simulink model "DrivetrainEv_3motor"  (R2019b)
settings: configuration reference "Reference" (kept outside this file)
undefined symbols (not defined in the file): b, b_CG, br, g, k, Mass, Ndiff_rear, NF, NR, T
libraries: autolibshared x8, autolibsharedcoupling x5, autolibcoupling x2, autolibutils x2, autolibshareddiff x1
(part 1 of 4)
settings Model: DataDictionary=SystemDD.sldd  ModifiedByFormat=The MathWorks, Inc.  PauseTimes=10  Creator=The MathWorks, Inc.  LastModifiedBy=The MathWorks, Inc.
settings ConfigSetRef: SourceName=Reference

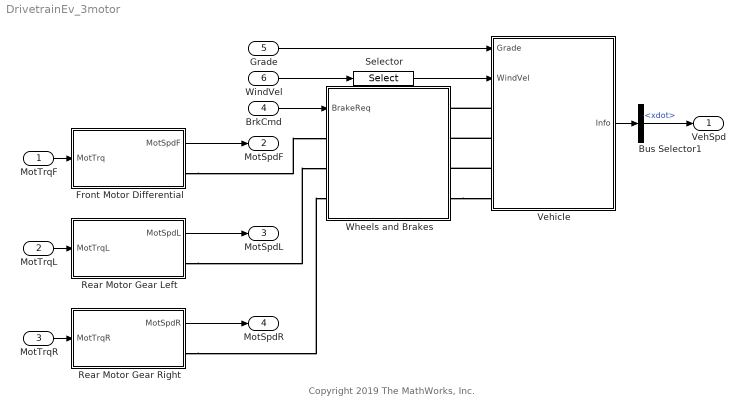
== system DrivetrainEv_3motor ==
  note: Copyright 2019 The MathWorks, Inc.
  MotTrqF : Inport
  MotTrqL : Inport  Port=2
  MotTrqR : Inport  Port=3
  BrkCmd : Inport  Port=4
  Grade : Inport  Port=5
  WindVel : Inport  Port=6
  Bus Selector1 : BusSelector  OutputSignals=BdyFrm.Cg.Vel.xdot
  Front Motor Differential : Subsystem  VariantControl=0
  Rear Motor Gear Left : Subsystem  VariantControl=0
  Rear Motor Gear Right : Subsystem  VariantControl=0
  Selector : Selector  InputPortWidth=3  IndexOptions=Index vector (dialog)  Indices=[1]  OutputSizes=1
  Vehicle : Subsystem
  Wheels and Brakes : Subsystem  VariantControlMode=Label  Variant=on  LabelModeActiveChoice=2
  VehSpd : Outport  VectorParamsAs1DForOutWhenUnconnected=off
  MotSpdF : Outport  Port=2  VectorParamsAs1DForOutWhenUnconnected=off  BusOutputAsStruct=on
  MotSpdL : Outport  Port=3  VectorParamsAs1DForOutWhenUnconnected=off  BusOutputAsStruct=on
  MotSpdR : Outport  Port=4  VectorParamsAs1DForOutWhenUnconnected=off  BusOutputAsStruct=on
  wires:
  Rear Motor Gear Left/1(MotSpdL) -> MotSpdL/1
  Rear Motor Gear Right/1(MotSpdR) -> MotSpdR/1
  MotTrqL/1 -> Rear Motor Gear Left/1(MotTrqL)
  MotTrqR/1 -> Rear Motor Gear Right/1(MotTrqR)
  WindVel/1 -> Selector/1
  BrkCmd/1 -> Wheels and Brakes/1(BrakeReq)
  Grade/1 -> Vehicle/1(Grade)
  Bus Selector1/1 -> VehSpd/1  "<xdot>"
  Vehicle/1(Info) -> Bus Selector1/1
  Selector/1 -> Vehicle/2(WindVel)
  Front Motor Differential/1(MotSpdF) -> MotSpdF/1
  MotTrqF/1 -> Front Motor Differential/1(MotTrq)
  connections:
  Front Motor Differential/RConn1 -- Wheels and Brakes/LConn1
  Vehicle/LConn1 -- Wheels and Brakes/RConn1
  Vehicle/LConn2 -- Wheels and Brakes/RConn2
  Vehicle/LConn3 -- Wheels and Brakes/RConn3
  Rear Motor Gear Left/RConn1 -- Wheels and Brakes/LConn2
  Rear Motor Gear Right/RConn1 -- Wheels and Brakes/LConn3
  Wheels and Brakes/RConn4 -- Vehicle/LConn4

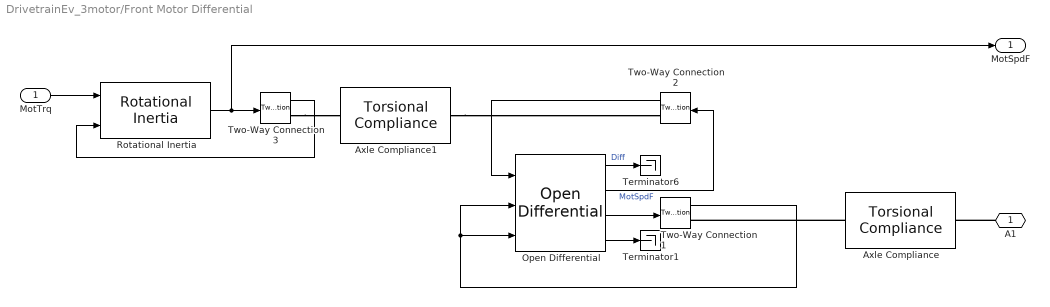
== system DrivetrainEv_3motor/Front Motor Differential ==
  MotTrq : Inport
  Axle Compliance : autolibsharedcoupling/Torsional Compliance  port_config=Two-way connection  extInfo=off  k=k  b=b  theta_o=theta_o  domega_o=domega_o  omega_c=omega_c  blkID=0  aMode=1
      settings: SourceProductName=Powertrain Blockset
  Axle Compliance1 : autolibsharedcoupling/Torsional Compliance  port_config=Two-way connection  extInfo=off  k=k  b=b  theta_o=theta_o  domega_o=domega_o  omega_c=omega_c  blkID=0  aMode=1
      settings: SourceProductName=Powertrain Blockset
  Open Differential : autolibshareddiff/Open Differential  DiffEffModelPopup=Constant  InterpMethod=Linear point-slope  extTamb=off  shaftSwitchMask=To the left of center-line  Ndiff=Ndiff_front  Jd=Jd  bd=bd  Jw1=Jw1  bw1=bw1  Jw2=Jw2  bw2=bw2  omegaw1o=omegaw1o  omegaw2o=omegaw2o  eta=1  eta_tbl=reshape([0.64 0.76 0.8 0.81 0.83 0.84 0.84 0.56 0.73 0.78 0.8 0.83 0.84 0.84 0.54 0.71 0.77 0.8 0.82 0.84 0.84 0.53 0.71 0.77 0.8 0.83 0.84 0.84 0.51 0.71 0.77 0.8 0.83 0.84 0.85 0.52 0.7 0.77 0.8 0.83 0.84 0.85 0.51 0.71 0.76 0.79 0.83 0.84 0.85 0.5 0.69 0.76 0.79 0.82 0.84 0.85 0.45 0.68 0.75 0.78 0.82 0.84 0.85 0.43 0.67 0.74 0.78 0.81 0.83 0.84 0.38 0.63 0.71 0.75 0.8 0.82 0.83 0.81 0.86 0.88 0.89 0.89 0.89 0.9 0.77 0.85 0.87 0.88 0.89 0.9 0.9 0.72 0.82 0.86 0.87 0.88 0.89 0.9 0.68 0.8 0.84 0.86 0.88 0.89 0.89 0.67 0.8 0.84 0.86 0.88 0.89 0.9 0.67 0.8 0.84 0.86 0.88 0.89 0.9 0.65 0.8 0.84 0.86 0.88 0.89 0.9 0.64 0.79 0.83 0.86 0.88 0.89 0.9 0.63 0.78 0.83 0.86 0.88 0.89 0.9 0.59 0.76 0.82 0.85 0.87 0.89 0.9 0.53 0.73 0.8 0.83 0.86 0.88 0.89], 7, 11, 2)  Trq_bpts=[25, 50, 75, 100, 150, 200, 250]  omega_bpts=[52.4 78.5 105 131 157 183 209 262 314 419 524]  Temp_bpts=[290 358]  Tamb=297.15  maxAbsSpd=5e3  aMode=1
      settings: SourceProductName=Powertrain Blockset
  Rotational Inertia : autolibsharedcoupling/Rotational Inertia  port_config=Simulink  extInfo=off  externJ=off  J=.01  b=.001  omega_o=0  blkID=0  aMode=1
      settings: SourceProductName=Powertrain Blockset  SourceProductBaseCode=PW
  Terminator1 : Terminator
  Terminator6 : Terminator
  Two-Way Connection1 : TwoWayConnection
  Two-Way Connection2 : TwoWayConnection
  Two-Way Connection3 : TwoWayConnection
  A1 : PMIOPort  Side=Right
  MotSpdF : Outport  VectorParamsAs1DForOutWhenUnconnected=off
  wires:
  Open Differential/2 -> Two-Way Connection2/1  "MotSpdF"
  Open Differential/3 -> Two-Way Connection1/1
  Two-Way Connection1/1 -> Open Differential/3, Open Differential/2
  Open Differential/1 -> Terminator6/1  "Diff"
  Open Differential/4 -> Terminator1/1
  Two-Way Connection2/1 -> Open Differential/1
  Rotational Inertia/1 -> MotSpdF/1, Two-Way Connection3/1
  MotTrq/1 -> Rotational Inertia/1
  Two-Way Connection3/1 -> Rotational Inertia/2
  connections:
  Axle Compliance/LConn1 -- Two-Way Connection1/RConn1
  A1/RConn1 -- Axle Compliance/RConn1
  Axle Compliance1/RConn1 -- Two-Way Connection2/RConn1
  Two-Way Connection3/RConn1 -- Axle Compliance1/LConn1

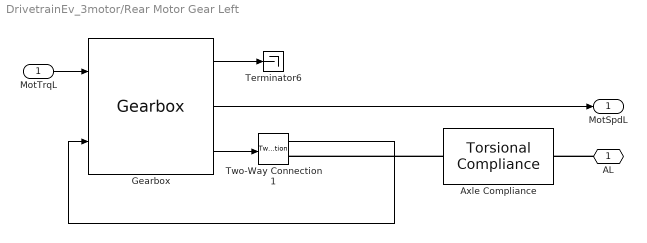
== system DrivetrainEv_3motor/Rear Motor Gear Left ==
  MotTrqL : Inport
  Axle Compliance : autolibsharedcoupling/Torsional Compliance  port_config=Two-way connection  extInfo=off  k=k  b=b  theta_o=theta_o  domega_o=domega_o  omega_c=omega_c  blkID=0  aMode=1
      settings: SourceProductName=Powertrain Blockset
  Gearbox : autolibcoupling/Gearbox  port_config=Simulink  input_config=Torque input - velocity output  DiffEffModelPopup=Constant  InterpMethod=Flat  dirSwitch=on  extTamb=off  N=Ndiff_rear  J1=J1  J2=J2  b1=b1_g  b2=b2_g  theta1_o=0  w1_o=w1_o  eta=1  eta_tbl=reshape([0.64 0.76 0.8 0.81 0.83 0.84 0.84 0.56 0.73 0.78 0.8 0.83 0.84 0.84 0.54 0.71 0.77 0.8 0.82 0.84 0.84 0.53 0.71 0.77 0.8 0.83 0.84 0.84 0.51 0.71 0.77 0.8 0.83 0.84 0.85 0.52 0.7 0.77 0.8 0.83 0.84 0.85 0.51 0.71 0.76 0.79 0.83 0.84 0.85 0.5 0.69 0.76 0.79 0.82 0.84 0.85 0.45 0.68 0.75 0.78 0.82 0.84 0.85 0.43 0.67 0.74 0.78 0.81 0.83 0.84 0.38 0.63 0.71 0.75 0.8 0.82 0.83 0.81 0.86 0.88 0.89 0.89 0.89 0.9 0.77 0.85 0.87 0.88 0.89 0.9 0.9 0.72 0.82 0.86 0.87 0.88 0.89 0.9 0.68 0.8 0.84 0.86 0.88 0.89 0.89 0.67 0.8 0.84 0.86 0.88 0.89 0.9 0.67 0.8 0.84 0.86 0.88 0.89 0.9 0.65 0.8 0.84 0.86 0.88 0.89 0.9 0.64 0.79 0.83 0.86 0.88 0.89 0.9 0.63 0.78 0.83 0.86 0.88 0.89 0.9 0.59 0.76 0.82 0.85 0.87 0.89 0.9 0.53 0.73 0.8 0.83 0.86 0.88 0.89], 7, 11, 2)  Trq_bpts=[25, 50, 75, 100, 150, 200, 250]  omega_bpts=[52.4 78.5 105 131 157 183 209 262 314 419 524]  Temp_bpts=[290 358]  Tamb=297.15  blkID=0
      settings: SourceProductName=Powertrain Blockset  SourceProductBaseCode=PW
  Terminator6 : Terminator
  Two-Way Connection1 : TwoWayConnection
  AL : PMIOPort  Side=Right
  MotSpdL : Outport  VectorParamsAs1DForOutWhenUnconnected=off
  wires:
  Gearbox/2 -> MotSpdL/1
  MotTrqL/1 -> Gearbox/1
  Gearbox/3 -> Two-Way Connection1/1
  Two-Way Connection1/1 -> Gearbox/2
  Gearbox/1 -> Terminator6/1
  connections:
  Axle Compliance/LConn1 -- Two-Way Connection1/RConn1
  AL/RConn1 -- Axle Compliance/RConn1

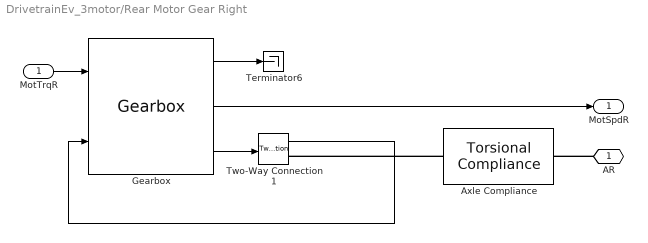
== system DrivetrainEv_3motor/Rear Motor Gear Right ==
  MotTrqR : Inport
  Axle Compliance : autolibsharedcoupling/Torsional Compliance  port_config=Two-way connection  extInfo=off  k=k  b=b  theta_o=theta_o  domega_o=domega_o  omega_c=omega_c  blkID=0  aMode=1
      settings: SourceProductName=Powertrain Blockset
  Gearbox : autolibcoupling/Gearbox  port_config=Simulink  input_config=Torque input - velocity output  DiffEffModelPopup=Constant  InterpMethod=Flat  dirSwitch=on  extTamb=off  N=Ndiff_rear  J1=J1  J2=J2  b1=b1_g  b2=b2_g  theta1_o=0  w1_o=w1_o  eta=1  eta_tbl=reshape([0.64 0.76 0.8 0.81 0.83 0.84 0.84 0.56 0.73 0.78 0.8 0.83 0.84 0.84 0.54 0.71 0.77 0.8 0.82 0.84 0.84 0.53 0.71 0.77 0.8 0.83 0.84 0.84 0.51 0.71 0.77 0.8 0.83 0.84 0.85 0.52 0.7 0.77 0.8 0.83 0.84 0.85 0.51 0.71 0.76 0.79 0.83 0.84 0.85 0.5 0.69 0.76 0.79 0.82 0.84 0.85 0.45 0.68 0.75 0.78 0.82 0.84 0.85 0.43 0.67 0.74 0.78 0.81 0.83 0.84 0.38 0.63 0.71 0.75 0.8 0.82 0.83 0.81 0.86 0.88 0.89 0.89 0.89 0.9 0.77 0.85 0.87 0.88 0.89 0.9 0.9 0.72 0.82 0.86 0.87 0.88 0.89 0.9 0.68 0.8 0.84 0.86 0.88 0.89 0.89 0.67 0.8 0.84 0.86 0.88 0.89 0.9 0.67 0.8 0.84 0.86 0.88 0.89 0.9 0.65 0.8 0.84 0.86 0.88 0.89 0.9 0.64 0.79 0.83 0.86 0.88 0.89 0.9 0.63 0.78 0.83 0.86 0.88 0.89 0.9 0.59 0.76 0.82 0.85 0.87 0.89 0.9 0.53 0.73 0.8 0.83 0.86 0.88 0.89], 7, 11, 2)  Trq_bpts=[25, 50, 75, 100, 150, 200, 250]  omega_bpts=[52.4 78.5 105 131 157 183 209 262 314 419 524]  Temp_bpts=[290 358]  Tamb=297.15  blkID=0
      settings: SourceProductName=Powertrain Blockset  SourceProductBaseCode=PW
  Terminator6 : Terminator
  Two-Way Connection1 : TwoWayConnection
  AR : PMIOPort  Side=Right
  MotSpdR : Outport  VectorParamsAs1DForOutWhenUnconnected=off
  wires:
  Gearbox/1 -> Terminator6/1
  Two-Way Connection1/1 -> Gearbox/2
  Gearbox/3 -> Two-Way Connection1/1
  MotTrqR/1 -> Gearbox/1
  Gearbox/2 -> MotSpdR/1
  connections:
  AR/RConn1 -- Axle Compliance/RConn1
  Axle Compliance/LConn1 -- Two-Way Connection1/RConn1

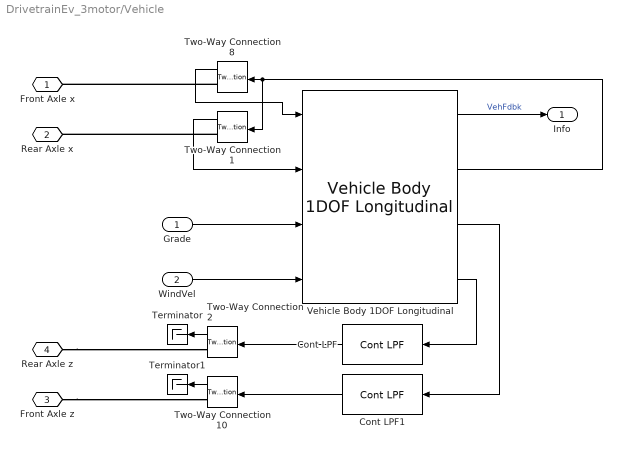
== system DrivetrainEv_3motor/Vehicle ==
  Grade : Inport
  WindVel : Inport  Port=2
  Cont LPF : autolibutils/Cont LPF  wc=wc  aMode=aMode
      settings: SourceProductName=Powertrain Blockset  SourceProductBaseCode=PW
  Cont LPF1 : autolibutils/Cont LPF  wc=wc  aMode=aMode
      settings: SourceProductName=Powertrain Blockset  SourceProductBaseCode=PW
  Terminator : Terminator
  Terminator1 : Terminator
  Two-Way Connection{1..2,8,10} (4 alike) : TwoWayConnection
  Vehicle Body 1DOF Longitudinal : autolibshared/Vehicle Body 1DOF Longitudinal  VariantControl=SL  extFMode=off  extMMode=off  extTamb=off  wind3D=off  aMode=1  NF=NF  NR=NR  m=Mass  a=a_CG  b=b_CG  h=h  Cd=Cd  Cl=0  Cpm=0  Af=Af  x_o=x_o  xdot_o=xdot_o  Pabs=Pabs  T=T  g=g
      settings: SourceProductName=Powertrain Blockset  SourceProductBaseCode=PW
  Front Axle x : PMIOPort  Side=Left
  Rear Axle x : PMIOPort  Port=2  Side=Left
  Front Axle z : PMIOPort  Port=3  Side=Left
  Rear Axle z : PMIOPort  Port=4  Side=Left
  Info : Outport  VectorParamsAs1DForOutWhenUnconnected=off
  wires:
  Vehicle Body 1DOF Longitudinal/3 -> Cont LPF1/1
  Vehicle Body 1DOF Longitudinal/2 -> Two-Way Connection1/1, Two-Way Connection8/1
  Two-Way Connection8/1 -> Vehicle Body 1DOF Longitudinal/1
  Vehicle Body 1DOF Longitudinal/1 -> Info/1  "VehFdbk"
  Two-Way Connection1/1 -> Vehicle Body 1DOF Longitudinal/2
  Vehicle Body 1DOF Longitudinal/4 -> Cont LPF/1
  Grade/1 -> Vehicle Body 1DOF Longitudinal/3
  WindVel/1 -> Vehicle Body 1DOF Longitudinal/4
  Cont LPF/1 -> Two-Way Connection2/1
  Cont LPF1/1 -> Two-Way Connection10/1
  Two-Way Connection2/1 -> Terminator/1
  Two-Way Connection10/1 -> Terminator1/1
  connections:
  Two-Way Connection8/RConn1 -- Front Axle x/RConn1
  Front Axle z/RConn1 -- Two-Way Connection10/RConn1
  Two-Way Connection1/RConn1 -- Rear Axle x/RConn1
  Rear Axle z/RConn1 -- Two-Way Connection2/RConn1

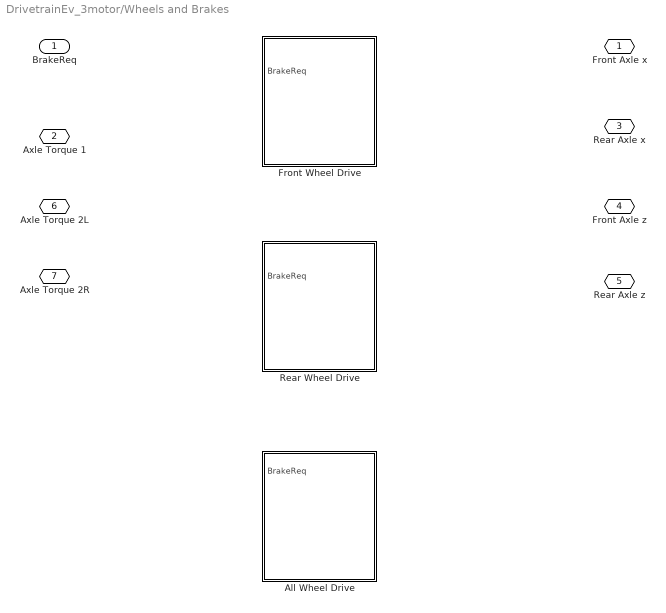
== system DrivetrainEv_3motor/Wheels and Brakes ==
  BrakeReq : Inport
  All Wheel Drive : Subsystem  VariantControl=2
  Front Wheel Drive : Subsystem  VariantControl=0
  Rear Wheel Drive : Subsystem  VariantControl=1
  Front Axle x : PMIOPort  Side=Right
  Axle Torque 1 : PMIOPort  Port=2  Side=Left
  Rear Axle x : PMIOPort  Port=3  Side=Right
  Front Axle z : PMIOPort  Port=4  Side=Right
  Rear Axle z : PMIOPort  Port=5  Side=Right
  Axle Torque 2L : PMIOPort  Port=6  Side=Left
  Axle Torque 2R : PMIOPort  Port=7  Side=Left
